simulink model "ex_11_1"  (R2021b)
settings: Solver=ode45  StartTime=0.0  StopTime=2.0  RelTol=1e-3  EnableMultiTasking=on
settings Model: Creator=Yuantao  LastModifiedBy=Yuantao
settings SolverCC: AlgebraicLoopSolver=TrustRegion
settings DataIOCC: LimitDataPoints=on  SaveFormat=Array  SignalLoggingSaveFormat=ModelDataLogs  ReturnWorkspaceOutputs=off
settings OptimizationCC: InitFltsAndDblsToZero=on  LifeSpan=inf
settings DebuggingCC: SaveWithParameterizedLinksMsg=none  UnderspecifiedInitializationDetection=Classic  MergeDetectMultiDrivingBlocksExec=none  SignalResolutionControl=TryResolveAllWithWarning  MultiTaskDSMMsg=warning  MultiTaskCondExecSysMsg=none  FcnCallInpInsideContextMsg=warning  SFUnexpectedBacktrackingDiag=warning  SFNoUnconditionalDefaultTransitionDiag=warning  SFExecutionAtInitializationDiag=none  SFMachineParentedDataDiag=warning  ArithmeticOperatorsInVariantConditions=warning
settings HardwareCC: ProdBitPerPointer=32  ProdBitPerSizeT=32  ProdBitPerPtrDiffT=32  ProdLargestAtomicFloat=None  ProdIntDivRoundTo=Undefined  ProdEndianess=Unspecified  ProdWordSize=32  ProdHWDeviceType=32-bit Generic
settings ModelReferenceCC: PropagateSignalLabelsOutOfModel=off
settings SFSimCC: SimParseCustomCode=off
settings CodeAppCC: StateflowObjectComments=on
settings GRTTargetCC: TargetFcnLib=ansi_tfl_tmw.mat  TargetLangStandard=C89/C90 (ANSI)  CombineOutputUpdateFcns=off  GRTInterface=on
settings ConfigComp: CovMetricSettings=dw  CovSaveCumulativeToWorkspaceVar=on  CovSaveSingleToWorkspaceVar=on

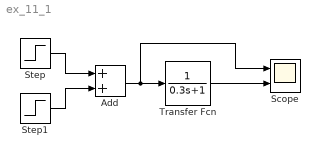
== system ex_11_1 ==
  Add : Sum
  Scope : Scope  NumInputPorts=2
  Step : Step  StopFcn=disp('stoped!')  Time=0  SampleTime=0
  Step1 : Step  StopFcn=disp('stoped!')  Time=0.5  After=-1  SampleTime=0
  Transfer Fcn : TransferFcn  Denominator=[0.3 1]
  wires:
  Transfer Fcn/1 -> Scope/2
  Add/1 -> Transfer Fcn/1, Scope/1
  Step/1 -> Add/1
  Step1/1 -> Add/2
